simulink model "MultirotorSimPx4v1_8FPHTFullGainMatrix"  (R2020b)
settings: Solver=VariableStepAuto  StartTime=0.0  StopTime=Simulation.T_END  MaxStep=Simulation.TS_MAX  RelTol=1e-3  EnableMultiTasking=on
PreLoadFcn:
  | % InitializeParameters;
undefined symbols (not defined in the file): Aero, Ctrl, Initial, Motor, Uav, Wind
libraries: QuaternionLibrary x10, simulink_extras x2, cstblocks x1
(part 1 of 2)
settings Model: Creator=jban039  LastModifiedBy=jeremie
settings DataIOCC: Decimation=10  ExternalInput=getinputstruct(op1(2))  InitialState=getstatestruct(op)  SaveFormat=StructureWithTime  OutputTimes=Simulation.T_OUT
settings OptimizationCC: LifeSpan=inf
settings DebuggingCC: ReadBeforeWriteMsg=DisableAll  WriteAfterWriteMsg=DisableAll  WriteAfterReadMsg=DisableAll  MultiTaskDSMMsg=none  UnconnectedLineMsg=none  AllowSymbolicDim=off  SFUnexpectedBacktrackingDiag=warning  SFNoUnconditionalDefaultTransitionDiag=warning  SFExecutionAtInitializationDiag=none  ArithmeticOperatorsInVariantConditions=warning
settings ModelReferenceCC: UpdateModelReferenceTargets=IfOutOfDate  ModelReferenceMinAlgLoopOccurrences=on  PropagateSignalLabelsOutOfModel=off
settings SFSimCC: SFSimEcho=off  SimUseLocalCustomCode=off  CustomCodeUndefinedFunction=UseInterfaceOnly
settings RTWCC: RTWUseLocalCustomCode=off
settings CodeAppCC: StateflowObjectComments=on
settings GRTTargetCC: TargetLangStandard=C89/C90 (ANSI)
settings ConfigComp: CovMetricSettings=dw  CovSaveCumulativeToWorkspaceVar=on  CovSaveSingleToWorkspaceVar=on  CovExternalEMLEnable=off

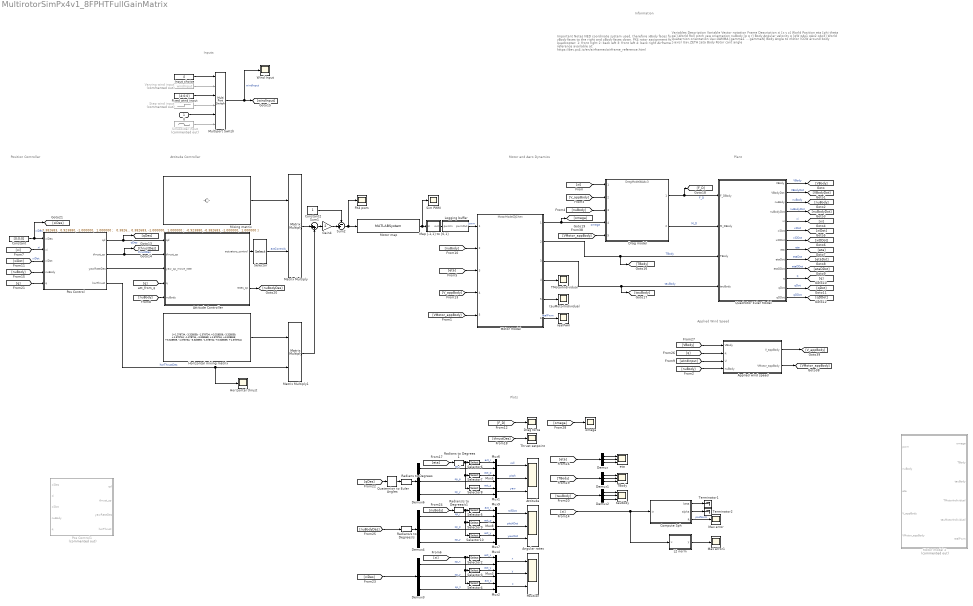
== system MultirotorSimPx4v1_8FPHTFullGainMatrix ==
  note: Plots
  note: Inputs
  note: Motor and Aero Dynamics
  note: Plant
  note: Attitude Controller
  note: Position Controller
  note: Applied Wind Speed
  note: Important Notes
      |
      | NED coordinate system used, therefore xBody faces forward, yBody faces to the right and zBody faces down.
      | PX4 rotor assignment for quadcopter:
      | 1: front right
      | 2: back left
      | 3: front left
      | 4: back right
      | Airframe reference available at:
      | https://dev.px4.io/en/airframes/airframe_reference.html
  note: Information
  note: Variables Description
      |
      | Variable
      | Vector notation
      | Frame
      | Description
      |
      | xi
      | [x y z]
      | World
      | Position
      |
      | eta
      | [phi theta psi]
      | World
      | Roll pitch yaw orientation
      |
      | nuBody
      | [p q r]
      | Body
      | Angular velocity
      |
      | q
      | [qW qAx1 qAx2 qAx3]
      | World
      | Quaternion orientation
      |
      | Uav.GAMMA
      | [gamma1 ... gammaN]
      | Body
      | Angle to motor (CCW around body z-axis)
      |
      | Uav.ZETA
      | zeta
      | Body
      | Rotor cant angle
  U : Inport  PortDimensions=3
  Angular rates : Scope  NumInputPorts=3
  Applied wind speed : Subsystem
  Attitude : Scope  NumInputPorts=3
  Attitude Controller : Subsystem
      mask Display: fprintf('MC_ATT_CONTROL\n\nCONTINUOUS')
  Compute Sph : MATLAB Function  TreatAsAtomicUnit=on
  Constant : Constant  Value=[0;0;0]
  Constant2 : Constant
  Demux{,1..4,6} (6 alike) : Demux  Outputs=3
  Drag force : Scope
  Drag model : ModelReference  ModelNameDialog=DragModelAIAAv3  SimulationMode=Normal  ModelReferenceVersion=5.2
  Fixed wind input : Constant  Value=[4;0;0]
  Gain4 : Gain  Gain=2
  Horizontal mixing matrix : Constant  Value=|
      | [+1.378734, -3.328559;
      |  -1.378734, +3.328559;
      |  -3.328559, +1.378734;
      |  -1.378734, -3.328559;
      |  +1.378734, +3.328559;
      |  +3.328559, -1.378734;
      |  -3.328559, -1.378734;
      |  +3.328559, +1.378734]
  Horizontal thrust : Scope
  Input choice : Constant  Value=4
  L2 norm : MATLAB Function  TreatAsAtomicUnit=on
  Logging buffer : Subsystem
  Map [-1,1] to [0,1] : Subsystem
  Matrix Multiply : Product  Multiplication=Matrix(*)
  Matrix Multiply1 : Product  Multiplication=Matrix(*)
  Max error : Scope
  Max error1 : Scope
  Mixing matrix : Constant  Value=|
      | [-0.382683,  0.923880, -1.000000,  1.000000 ;
      |   0.382683, -0.923880, -1.000000,  1.000000 ;
      |  -0.923880,  0.382683,  1.000000,  1.000000 ;
      |  -0.382683, -0.923880,  1.000000,  1.000000 ;
      |   0.382683,  0.923880,  1.000000,  1.000000 ;
      |   0.923880, -0.382683,  1.000000,  1.000000 ;
      |   0.923880,  0.382683, -1.000000,  1.000000 ;
      |  -0.923880, -0.382683, -1.000000,  1.000000 ]
  Motor map : MATLABSystem  System=MotorMap  airframeConfig=5  SimulateUsing=Code generation
      mask Type: MotorMap
      mask Display:
      | disp(['MOTOR' char(10) 'MAP' char(10) 'octa_x']);
      | port_label('input',1,'px4PWM');
      | port_label('output',1,'simPWM');
  Motor model : ModelReference  ModelNameDialog=MotorModelZJChen  SimulationMode=Normal  ModelReferenceVersion=5.6
  Motor model 2 : Subsystem  Commented=on
  Multiport Switch : MultiPortSwitch  Inputs=5
  Mux{1..9} (9 alike) : Mux  Inputs=2
  PX4 pwm : Scope
  Pos Control : Subsystem
      mask Display: fprintf('POS CONTROL\n\nFPHT\n\nCONTINUOUS')
  Pos Control1 : Subsystem  Commented=on
      mask Display: fprintf('POS CONTROL\n\nFPHT\n\nCONTINUOUS')
  Position : Scope  NumInputPorts=3
  Quadrotor Euler Model : Subsystem
  Quaternion to Euler Angles : QuaternionLibrary/Quaternion to Euler Angles
  "Radians to Degrees " : QuaternionLibrary/Radians to Degrees   SystemSampleTime=-1  VariantActivationTime=update diagram  Latency=0  AutoFrameSizeCalculation=off
  Radians to Degrees 1 : QuaternionLibrary/Radians to Degrees   SystemSampleTime=-1  VariantActivationTime=update diagram  Latency=0  AutoFrameSizeCalculation=off
  Radians/s to Degrees/s : QuaternionLibrary/Radians//s to Degrees//s  SystemSampleTime=-1  VariantActivationTime=update diagram  Latency=0  AutoFrameSizeCalculation=off
  Radians/s to Degrees/s1 : QuaternionLibrary/Radians//s to Degrees//s  SystemSampleTime=-1  VariantActivationTime=update diagram  Latency=0  AutoFrameSizeCalculation=off
  Selector : Selector  InputPortWidth=8  IndexOptions=Index vector (dialog)  Indices=[1:4]  OutputSizes=1
  Selector10 : Selector  InputPortWidth=3  IndexOptions=Index vector (dialog)  Indices=3  OutputSizes=1
  Selector2 : Selector  InputPortWidth=3  IndexOptions=Index vector (dialog)  Indices=1  OutputSizes=1
  Selector3 : Selector  InputPortWidth=3  IndexOptions=Index vector (dialog)  Indices=2  OutputSizes=1
  Selector4 : Selector  InputPortWidth=3  IndexOptions=Index vector (dialog)  Indices=3  OutputSizes=1
  Selector5 : Selector  InputPortWidth=3  IndexOptions=Index vector (dialog)  Indices=1  OutputSizes=1
  Selector6 : Selector  InputPortWidth=3  IndexOptions=Index vector (dialog)  Indices=1  OutputSizes=1
  Selector7 : Selector  InputPortWidth=3  IndexOptions=Index vector (dialog)  Indices=2  OutputSizes=1
  Selector8 : Selector  InputPortWidth=3  IndexOptions=Index vector (dialog)  Indices=3  OutputSizes=1
  Selector9 : Selector  InputPortWidth=3  IndexOptions=Index vector (dialog)  Indices=2  OutputSizes=1
  Sim PWM : Scope
  Sinusoidal input : Sin  Commented=on  Amplitude=Wind.Ampl  Bias=Wind.Bias  Frequency=Wind.Freq  SampleTime=0
  Step wind input : Step  Commented=on  Time=Wind.StepTime  Before=Wind.StepInit  After=Wind.StepFinal  SampleTime=0
  Sum1 : Sum  Inputs=|++
  Sum2 : Sum  Inputs=-+|
  TBody : Scope  NumInputPorts=3
  TMotorIndividual : Scope
  Terminator1 : Terminator
  Terminator2 : Terminator
  Thrust setpoint : Scope
  Varying wind input : FromWorkspace  Commented=on  VariableName=windInput
  Wind Input : Scope
  eta : Scope  NumInputPorts=3
  omega : Scope
  realPwm : Scope
  tauBody : Scope  NumInputPorts=3
  tauMotorIndividual : Scope
  wires:
  Motor model/1 -> Drag model/4, [omega]  "omega"
  Motor model/2 -> [TBody], Quadrotor Euler Model/3(TBody)  "TBody"
  Drag model/2 -> Quadrotor Euler Model/2(M_DBody)  "M_D"
  Quadrotor Euler Model/1(VBody) -> [VBody]  "VBody"
  Quadrotor Euler Model/2(VBodyDot) -> [VBodyDot]  "VBodyDot"
  Quadrotor Euler Model/3(nuBody) -> [nuBody]  "nuBody"
  Quadrotor Euler Model/4(nuBodyDot) -> [nuBodyDot]  "nuBodyDot"
  Quadrotor Euler Model/5(xi) -> [xi]  "xi"
  Quadrotor Euler Model/6(xiDot) -> [xiDot]  "xiDot"
  Quadrotor Euler Model/7(xiDDot) -> [xiDDot]  "xiDDot"
  Quadrotor Euler Model/8(eta) -> [eta]  "eta"
  Quadrotor Euler Model/9(etaDot) -> [etaDot]  "etaDot"
  Quadrotor Euler Model/10(etaDDot) -> [etaDDot]  "etaDDot"
  [V_appBody] -> Drag model/2
  [nuBody] -> Motor model/2
  Quadrotor Euler Model/11(q) -> [q]  "q"
  Quadrotor Euler Model/12(qDot) -> [qDot]  "qDot"
  Quadrotor Euler Model/13(qDDot) -> [qDDot]  "qDDot"
  Drag model/1 -> Quadrotor Euler Model/1(F_DBody), [F_D]  "F_D"
  Logging buffer/1(pwmOut) -> Motor model/1  "pwm"
  Sum2/1 -> PX4 pwm/1, Motor map/1
  [nuBody] -> Drag model/3
  [eta] -> Motor model/3
  [V_appBody] -> Motor model/4
  Motor model/4 -> TMotorIndividual/1
  Motor model/5 -> tauMotorIndividual/1
  [xi] -> Drag model/1
  [VMotor_appBody] -> Motor model/5
  [VMotor_appBody] -> Drag model/5
  Pos Control/1(qd) -> Attitude Controller/1(qd), [qDes]  "qDes"
  Motor model/3 -> [tauBody], Quadrotor Euler Model/4(tauBody)  "tauBody"
  [VBody] -> Applied wind speed/1(VBody)
  [q] -> Applied wind speed/2(q)
  [windInput] -> Applied wind speed/3(U)
  Applied wind speed/1(V_appBody) -> [V_appBody]
  Applied wind speed/2(VMotor_appBody) -> [VMotor_appBody]
  [nuBody] -> Applied wind speed/4(nuBody)
  Motor model/6 -> realPwm/1  "realPwm"
  [nuBody] -> Attitude Controller/5(nuBody)
  Motor map/1 -> Sim PWM/1, Map [-1,1] to [0,1]/1(in)
  Map [-1,1] to [0,1]/1(out) -> Logging buffer/1(pwmIn)
  Selector/1 -> Matrix Multiply/2  "actControls"
  Mixing matrix/1 -> Matrix Multiply/1
  Attitude Controller/1(actuators_control) -> Selector/1
  Gain4/1 -> Sum2/2
  Constant2/1 -> Sum2/1
  Matrix Multiply/1 -> Sum1/1
  Pos Control/2(thrust_sp) -> Attitude Controller/2(thrust_sp), [thrustDes]  "thrustDes"
  Pos Control/3(yawRateDes) -> Attitude Controller/3(yaw_sp_move_rate)
  [xiDot] -> Pos Control/3(xiDot)  "xiDot"
  [xi] -> Pos Control/2(xi)  "xi"
  [nuBody] -> Pos Control/4(nuBody)
  Constant/1 -> [xiDes], Pos Control/1(xiDes)  "xiDes"
  Attitude Controller/2(rates_sp) -> [nuBodyDes]
  Matrix Multiply1/1 -> Sum1/2
  Horizontal mixing matrix/1 -> Matrix Multiply1/1
  Pos Control/4(horThrust) -> Horizontal thrust/1, Matrix Multiply1/2  "horThrustDes"
  [q] -> Attitude Controller/4(q)
  [q] -> Pos Control/5(q)
  Sum1/1 -> Gain4/1
  Mux7/1 -> Angular rates/3  "yawDot"
  [nuBody] -> Radians/s to Degrees/s1/1
  Radians/s to Degrees/s1/1 -> Selector5/1, Selector9/1, Selector10/1
  Radians/s to Degrees/s/1 -> Demux4/1
  Mux8/1 -> Angular rates/2  "pitchDot"
  Mux9/1 -> Angular rates/1  "rollDot"
  Selector10/1 -> Mux7/1  "act_y"
  Demux4/2 -> Mux8/2  "sp_p"
  Demux4/1 -> Mux9/2  "sp_r"
  [nuBodyDes] -> Radians/s to Degrees/s/1
  Selector9/1 -> Mux8/1  "act_p"
  Selector5/1 -> Mux9/1  "act_r"
  Demux4/3 -> Mux7/2  "sp_y"
  Mux2/1 -> Position/3  "z"
  [xi] -> Selector2/1, Selector3/1, Selector4/1
  [xiDes] -> Demux3/1
  Mux3/1 -> Position/2  "y"
  Mux4/1 -> Position/1  "x"
  Selector4/1 -> Mux2/1  "act_z"
  Demux3/2 -> Mux3/2  "sp_y"
  Demux3/1 -> Mux4/2  "sp_x"
  Selector3/1 -> Mux3/1  "act_y"
  Selector2/1 -> Mux4/1  "act_x"
  Demux3/3 -> Mux2/2  "sp_z"
  L2 norm/1(y) -> Max error1/1
  [F_D] -> Drag force/1
  Compute Sph/3(R) -> Max error/1  "posNorm"
  Compute Sph/2(alpha) -> Terminator2/1
  Compute Sph/1(beta) -> Terminator1/1
  Demux2/3 -> tauBody/3
  Demux2/2 -> tauBody/2
  [tauBody] -> Demux2/1
  Demux2/1 -> tauBody/1
  Demux1/1 -> TBody/1
  [TBody] -> Demux1/1
  Demux1/2 -> TBody/2
  Demux1/3 -> TBody/3
  [thrustDes] -> Thrust setpoint/1
  Demux6/3 -> Mux1/2  "sp_y"
  Selector6/1 -> Mux6/1  "act_r"
  Selector7/1 -> Mux5/1  "act_p"
  Quaternion to Euler Angles/1 -> "Radians to Degrees "/1
  Demux6/1 -> Mux6/2  "sp_r"
  Demux6/2 -> Mux5/2  "sp_p"
  Selector8/1 -> Mux1/1  "act_y"
  [qDes] -> Quaternion to Euler Angles/1
  Mux6/1 -> Attitude/1  "roll"
  Mux5/1 -> Attitude/2  "pitch"
  "Radians to Degrees "/1 -> Demux6/1
  Radians to Degrees 1/1 -> Selector8/1, Selector7/1, Selector6/1
  [eta] -> Radians to Degrees 1/1
  Mux1/1 -> Attitude/3  "yaw"
  Demux/3 -> eta/3
  Demux/2 -> eta/2
  Demux/1 -> eta/1
  [eta] -> Demux/1
  [xi] -> Compute Sph/1(in), L2 norm/1(u)
  Sinusoidal input/1 -> Multiport Switch/6
  U/1 -> Multiport Switch/5
  Input choice/1 -> Multiport Switch/1
  Step wind input/1 -> Multiport Switch/4
  Multiport Switch/1 -> [windInput], Wind Input/1  "windInput"
  Fixed wind input/1 -> Multiport Switch/3
  Varying wind input/1 -> Multiport Switch/2
  [omega] -> omega/1

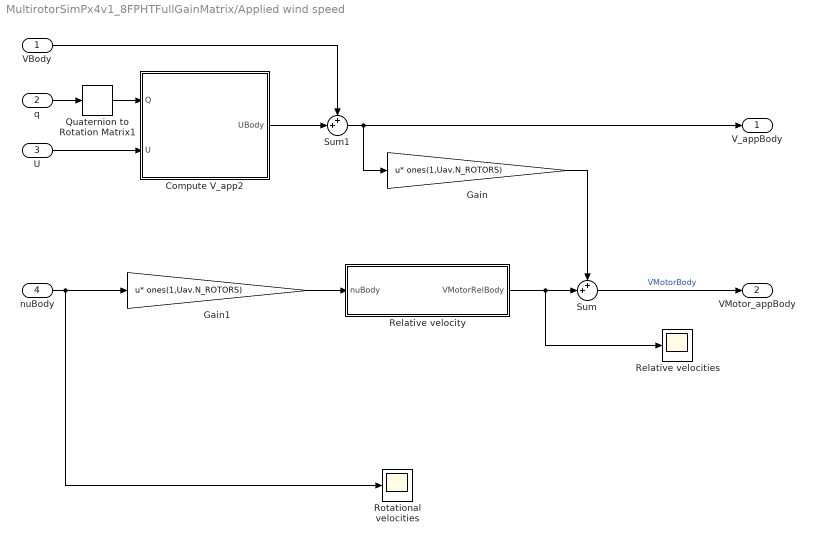
== system MultirotorSimPx4v1_8FPHTFullGainMatrix/Applied wind speed ==
  VBody : Inport  Unit=m/s
  q : Inport  Port=2
  U : Inport  Port=3  Unit=m/s
  nuBody : Inport  Port=4  Unit=rad/s
  Compute V_app2 : MATLAB Function  TreatAsAtomicUnit=on
  Gain : Gain  Gain=ones(1,Uav.N_ROTORS)  Multiplication=Matrix(u*K)
  Gain1 : Gain  Gain=ones(1,Uav.N_ROTORS)  Multiplication=Matrix(u*K)
  Quaternion to Rotation Matrix1 : QuaternionLibrary/Quaternion to Rotation Matrix
  Relative velocities : Scope
  Relative velocity : MATLAB Function  TreatAsAtomicUnit=on
  Rotational velocities : Scope
  Sum : Sum  Inputs=++|
  Sum1 : Sum  Inputs=++|
  V_appBody : Outport  Unit=m/s  VectorParamsAs1DForOutWhenUnconnected=off
  VMotor_appBody : Outport  Port=2  Unit=m/s  PortDimensions=[3,Uav.N_ROTORS]  VectorParamsAs1DForOutWhenUnconnected=off
  wires:
  U/1 -> Compute V_app2/2(U)
  Sum/1 -> VMotor_appBody/1  "VMotorBody"
  Quaternion to Rotation Matrix1/1 -> Compute V_app2/1(Q)
  nuBody/1 -> Gain1/1, Rotational velocities/1
  Gain/1 -> Sum/1
  VBody/1 -> Sum1/1
  q/1 -> Quaternion to Rotation Matrix1/1
  Relative velocity/1(VMotorRelBody) -> Relative velocities/1, Sum/2
  Compute V_app2/1(UBody) -> Sum1/2
  Sum1/1 -> Gain/1, V_appBody/1
  Gain1/1 -> Relative velocity/1(nuBody)

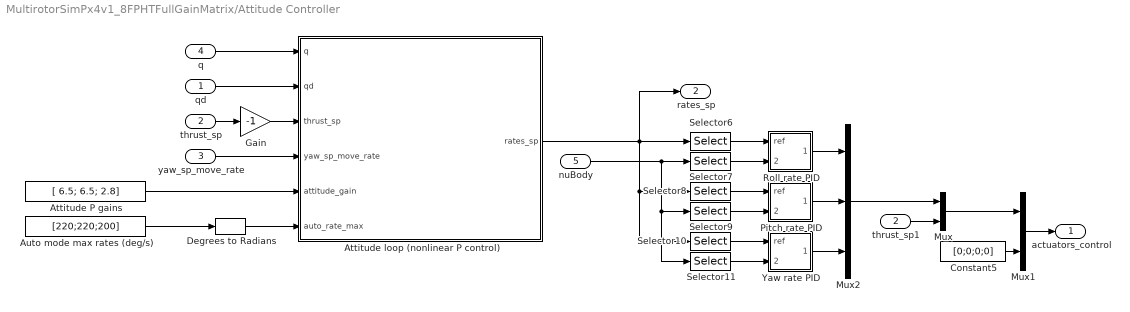
== system MultirotorSimPx4v1_8FPHTFullGainMatrix/Attitude Controller ==
  qd : Inport
  thrust_sp : Inport  Port=2  PortDimensions=1
  yaw_sp_move_rate : Inport  Port=3
  q : Inport  Port=4
  nuBody : Inport  Port=5
  Attitude P gains : Constant  Value=[ 6.5; 6.5; 2.8]
  Attitude loop (nonlinear P control) : MATLAB Function  TreatAsAtomicUnit=on
  Auto mode max rates (deg/s) : Constant  Value=[220;220;200]
  Constant5 : Constant  Value=[0;0;0;0]
  Degrees to Radians : simulink_extras/Transformations/Degrees to Radians
  Gain : Gain  Gain=-1
  Mux : Mux  Inputs=2
  Mux1 : Mux  Inputs=2
  Mux2 : Mux  Inputs=3
  Pitch rate PID : Subsystem  mask{PID_P=0.15, PID_I=0.05, PID_D=0.003, PID_FC=30, PID_I_STATENAME='AttRatePID_I_pitch', PID_D_STATENAME='AttRatePID_D_pitch'}
      mask prompts: PID_P "P gain"; PID_I "I gain"; PID_D "D gain"; PID_FC "D filter cutoff (Hz)"; PID_I_STATENAME "Integartor state name"; PID_D_STATENAME "D filter state name"
      mask DialogControl DescGroupVar Prompt: PID Controller with Second Order Derivative Filter
      mask DialogControl DescTextVar Prompt: The derivative gain is applied on the derivative of y rather than that of the error (r-y).
      mask Display:
      | disp('PID(s)')
      | port_label('input', 1, 'r')
      | port_label('input', 2, 'y')
      | text(1,0,'2^{nd}','horizontalAlignment','right','interpreter','tex','verticalAlignment','bottom')
  Roll rate PID : Subsystem  mask{PID_P=0.15, PID_I=0.05, PID_D=0.003, PID_FC=30, PID_I_STATENAME='AttRatePID_I_roll', PID_D_STATENAME='AttRatePID_D_roll'}
      mask prompts: PID_P "P gain"; PID_I "I gain"; PID_D "D gain"; PID_FC "D filter cutoff (Hz)"; PID_I_STATENAME "Integartor state name"; PID_D_STATENAME "D filter state name"
      mask DialogControl DescGroupVar Prompt: PID Controller with Second Order Derivative Filter
      mask DialogControl DescTextVar Prompt: The derivative gain is applied on the derivative of y rather than that of the error (r-y).
      mask Display:
      | disp('PID(s)')
      | port_label('input', 1, 'r')
      | port_label('input', 2, 'y')
      | text(1,0,'2^{nd}','horizontalAlignment','right','interpreter','tex','verticalAlignment','bottom')
  Selector10 : Selector  InputPortWidth=3  IndexOptions=Index vector (dialog)  Indices=3  OutputSizes=1
  Selector11 : Selector  InputPortWidth=3  IndexOptions=Index vector (dialog)  Indices=3  OutputSizes=1
  Selector6 : Selector  InputPortWidth=3  IndexOptions=Index vector (dialog)  Indices=1  OutputSizes=1
  Selector7 : Selector  InputPortWidth=3  IndexOptions=Index vector (dialog)  Indices=1  OutputSizes=1
  Selector8 : Selector  InputPortWidth=3  IndexOptions=Index vector (dialog)  Indices=2  OutputSizes=1
  Selector9 : Selector  InputPortWidth=3  IndexOptions=Index vector (dialog)  Indices=2  OutputSizes=1
  Yaw rate PID : Subsystem  mask{PID_P=0.2, PID_I=0.1, PID_D=0, PID_FC=30, PID_I_STATENAME='AttRatePID_I_yaw', PID_D_STATENAME='AttRatePID_D_yaw'}
      mask prompts: PID_P "P gain"; PID_I "I gain"; PID_D "D gain"; PID_FC "D filter cutoff (Hz)"; PID_I_STATENAME "Integartor state name"; PID_D_STATENAME "D filter state name"
      mask DialogControl DescGroupVar Prompt: PID Controller with Second Order Derivative Filter
      mask DialogControl DescTextVar Prompt: The derivative gain is applied on the derivative of y rather than that of the error (r-y).
      mask Display:
      | disp('PID(s)')
      | port_label('input', 1, 'r')
      | port_label('input', 2, 'y')
      | text(1,0,'2^{nd}','horizontalAlignment','right','interpreter','tex','verticalAlignment','bottom')
  thrust_sp1 : InportShadow  Port=2  PortDimensions=1
  actuators_control : Outport  PortDimensions=8  VectorParamsAs1DForOutWhenUnconnected=off
  rates_sp : Outport  Port=2  VectorParamsAs1DForOutWhenUnconnected=off
  wires:
  thrust_sp1/1 -> Mux/2
  Gain/1 -> Attitude loop (nonlinear P control)/3(thrust_sp)
  Attitude loop (nonlinear P control)/1(rates_sp) -> rates_sp/1, Selector10/1, Selector8/1, Selector6/1
  thrust_sp/1 -> Gain/1
  Mux1/1 -> actuators_control/1
  Constant5/1 -> Mux1/2
  Mux/1 -> Mux1/1
  yaw_sp_move_rate/1 -> Attitude loop (nonlinear P control)/4(yaw_sp_move_rate)
  Degrees to Radians/1 -> Attitude loop (nonlinear P control)/6(auto_rate_max)
  Auto mode max rates (deg/s)/1 -> Degrees to Radians/1
  Attitude P gains/1 -> Attitude loop (nonlinear P control)/5(attitude_gain)
  q/1 -> Attitude loop (nonlinear P control)/1(q)
  qd/1 -> Attitude loop (nonlinear P control)/2(qd)
  Yaw rate PID/1(Out) -> Mux2/3
  Roll rate PID/1(Out) -> Mux2/1
  Pitch rate PID/1(Out) -> Mux2/2
  Mux2/1 -> Mux/1
  Selector6/1 -> Roll rate PID/1(ref)
  Selector7/1 -> Roll rate PID/2(meas)
  Selector8/1 -> Pitch rate PID/1(ref)
  Selector10/1 -> Yaw rate PID/1(ref)
  Selector11/1 -> Yaw rate PID/2(meas)
  Selector9/1 -> Pitch rate PID/2(meas)
  nuBody/1 -> Selector11/1, Selector9/1, Selector7/1

== system MultirotorSimPx4v1_8FPHTFullGainMatrix/Logging buffer ==
  pwmIn : Inport
  pwmOut : Outport  VectorParamsAs1DForOutWhenUnconnected=off
  wires:
  pwmIn/1 -> pwmOut/1

== system MultirotorSimPx4v1_8FPHTFullGainMatrix/Map [-1,1] to [0,1] ==
  in : Inport
  Constant : Constant
  Gain4 : Gain  Gain=0.5
  Sum : Sum  Inputs=++|
  out : Outport  VectorParamsAs1DForOutWhenUnconnected=off
  wires:
  Sum/1 -> Gain4/1
  Gain4/1 -> out/1
  in/1 -> Sum/2
  Constant/1 -> Sum/1

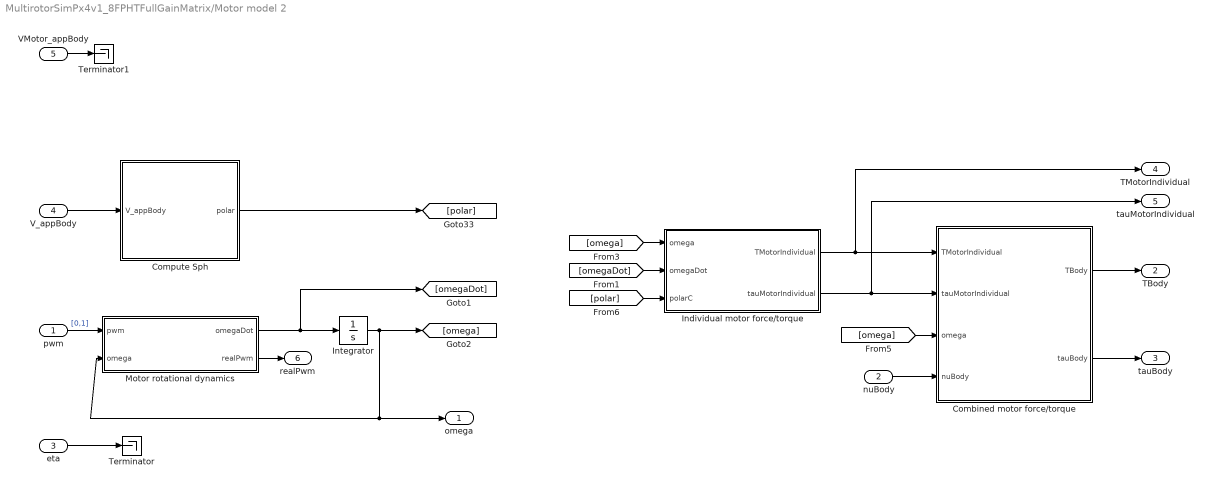
== system MultirotorSimPx4v1_8FPHTFullGainMatrix/Motor model 2 ==
  pwm : Inport  PortDimensions=Uav.N_ROTORS
  nuBody : Inport  Port=2  Unit=rad/s  PortDimensions=3
  eta : Inport  Port=3  Unit=rad  PortDimensions=3
  V_appBody : Inport  Port=4  Unit=m/s  PortDimensions=3
  VMotor_appBody : Inport  Port=5  Unit=m/s  PortDimensions=[3,Uav.N_ROTORS]
  Combined motor force/torque : MATLAB Function  TreatAsAtomicUnit=on
  Compute Sph : MATLAB Function  TreatAsAtomicUnit=on
  Individual motor force/torque : MATLAB Function  TreatAsAtomicUnit=on
  Integrator : Integrator  InitialCondition=Initial.OMEGA  LimitOutput=on  LowerSaturationLimit=zeros(size(Initial.OMEGA))  ContinuousStateAttributes='omega'
  Motor rotational dynamics : MATLAB Function  TreatAsAtomicUnit=on
  Terminator : Terminator
  Terminator1 : Terminator
  omega : Outport  Unit=rad/s  VectorParamsAs1DForOutWhenUnconnected=off
  TBody : Outport  Port=2  Unit=N  VectorParamsAs1DForOutWhenUnconnected=off
  tauBody : Outport  Port=3  Unit=N*m  VectorParamsAs1DForOutWhenUnconnected=off
  TMotorIndividual : Outport  Port=4  Unit=N  PortDimensions=[3,Uav.N_ROTORS]  VectorParamsAs1DForOutWhenUnconnected=off
  tauMotorIndividual : Outport  Port=5  Unit=N  PortDimensions=[3,Uav.N_ROTORS]  VectorParamsAs1DForOutWhenUnconnected=off
  realPwm : Outport  Port=6  VectorParamsAs1DForOutWhenUnconnected=off
  wires:
  [omegaDot] -> Individual motor force/torque/2(omegaDot)
  Compute Sph/1(polar) -> [polar]
  pwm/1 -> Motor rotational dynamics/1(pwm)  "[0,1]"
  [omega] -> Combined motor force/torque/3(omega)
  Combined motor force/torque/1(TBody) -> TBody/1
  [omega] -> Individual motor force/torque/1(omega)
  eta/1 -> Terminator/1
  V_appBody/1 -> Compute Sph/1(V_appBody)
  Individual motor force/torque/1(TMotorIndividual) -> Combined motor force/torque/1(TMotorIndividual), TMotorIndividual/1
  Motor rotational dynamics/1(omegaDot) -> [omegaDot], Integrator/1
  Integrator/1 -> [omega], Motor rotational dynamics/2(omega), omega/1
  Individual motor force/torque/2(tauMotorIndividual) -> tauMotorIndividual/1, Combined motor force/torque/2(tauMotorIndividual)
  nuBody/1 -> Combined motor force/torque/4(nuBody)
  Combined motor force/torque/2(tauBody) -> tauBody/1
  Motor rotational dynamics/2(realPwm) -> realPwm/1
  VMotor_appBody/1 -> Terminator1/1
  [polar] -> Individual motor force/torque/3(polarC)

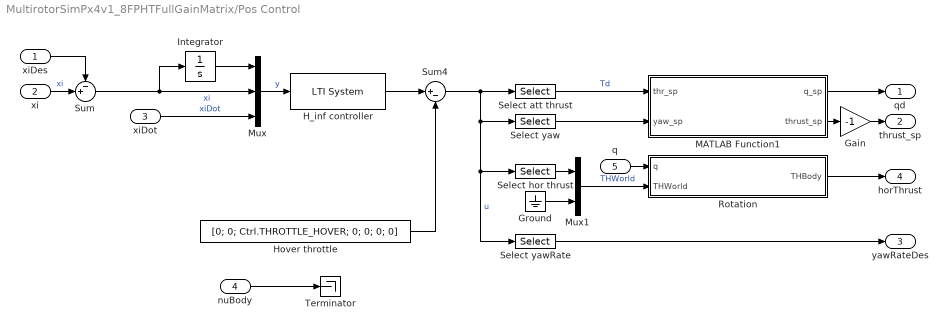
== system MultirotorSimPx4v1_8FPHTFullGainMatrix/Pos Control ==
  xiDes : Inport  Unit=m  PortDimensions=3
  xi : Inport  Port=2  Unit=m  PortDimensions=3
  xiDot : Inport  Port=3  Unit=m/s  PortDimensions=3
  nuBody : Inport  Port=4  Unit=rad/s
  q : Inport  Port=5
  Gain : Gain  Gain=-1
  Ground : Ground
  H_inf controller : cstblocks/LTI System  sys=Ctrl.K  IC=[]
  Hover throttle : Constant  Value=[0; 0; Ctrl.THROTTLE_HOVER; 0; 0; 0; 0]
  Integrator : Integrator
  MATLAB Function1 : MATLAB Function  TreatAsAtomicUnit=on
  Mux : Mux  Inputs=3
  Mux1 : Mux  Inputs=2
  Rotation : Subsystem
  Select att thrust : Selector  InputPortWidth=size(Ctrl.K.C, 1)  IndexOptions=Index vector (dialog)  Indices=[1:3]  OutputSizes=1
  Select hor thrust : Selector  InputPortWidth=size(Ctrl.K.C, 1)  IndexOptions=Index vector (dialog)  Indices=[4:5]  OutputSizes=1
  Select yaw : Selector  InputPortWidth=size(Ctrl.K.C, 1)  IndexOptions=Index vector (dialog)  Indices=[6]  OutputSizes=1
  Select yawRate : Selector  InputPortWidth=size(Ctrl.K.C, 1)  IndexOptions=Index vector (dialog)  Indices=[7]  OutputSizes=1
  Sum : Sum  Inputs=-+|
  Sum4 : Sum  Inputs=|+-
  Terminator : Terminator
  qd : Outport  VectorParamsAs1DForOutWhenUnconnected=off
  thrust_sp : Outport  Port=2  VectorParamsAs1DForOutWhenUnconnected=off
  yawRateDes : Outport  Port=3  Unit=rad/s  VectorParamsAs1DForOutWhenUnconnected=off
  horThrust : Outport  Port=4  PortDimensions=2  VectorParamsAs1DForOutWhenUnconnected=off
  wires:
  Select yawRate/1 -> yawRateDes/1
  nuBody/1 -> Terminator/1
  Rotation/1(THBody) -> horThrust/1
  Select yaw/1 -> MATLAB Function1/2(yaw_sp)
  MATLAB Function1/1(q_sp) -> qd/1
  MATLAB Function1/2(thrust_sp) -> Gain/1
  Select att thrust/1 -> MATLAB Function1/1(thr_sp)  "Td"
  Sum/1 -> Mux/2, Integrator/1  "xi"
  q/1 -> Rotation/1(q)
  Mux1/1 -> Rotation/2(THWorld)  "THWorld"
  Mux/1 -> H_inf controller/1  "y"
  Hover throttle/1 -> Sum4/2
  Sum4/1 -> Select yaw/1, Select yawRate/1, Select hor thrust/1, Select att thrust/1  "u"
  Gain/1 -> thrust_sp/1
  xiDes/1 -> Sum/1
  xi/1 -> Sum/2  "xi"
  Integrator/1 -> Mux/1
  xiDot/1 -> Mux/3  "xiDot"
  H_inf controller/1 -> Sum4/1
  Select hor thrust/1 -> Mux1/1
  Ground/1 -> Mux1/2

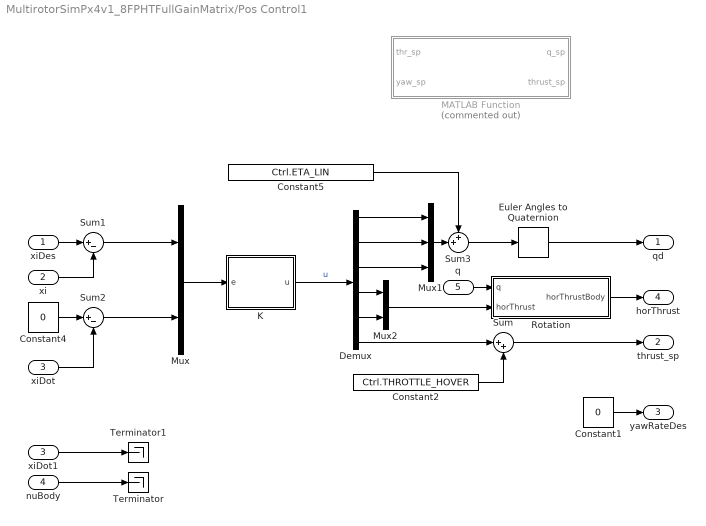
== system MultirotorSimPx4v1_8FPHTFullGainMatrix/Pos Control1 ==
  xiDes : Inport  Unit=m  PortDimensions=3
  xi : Inport  Port=2  Unit=m  PortDimensions=3
  xiDot : Inport  Port=3  Unit=m/s  PortDimensions=3
  nuBody : Inport  Port=4  Unit=rad/s
  q : Inport  Port=5
  Constant1 : Constant  Value=0
  Constant2 : Constant  Value=Ctrl.THROTTLE_HOVER
  Constant4 : Constant  Value=0
  Constant5 : Constant  Value=Ctrl.ETA_LIN
  Demux : Demux  Outputs=6
  Euler Angles to Quaternion : QuaternionLibrary/Euler Angles to Quaternion
  K : Subsystem
      mask Display:
      | text(0.5, 0.5, '\fontsize{30}K', 'horizontalAlignment', ...
      |     'center', 'verticalAlignment', 'middle', 'texmode', 'on')
  MATLAB Function : MATLAB Function  Commented=on  TreatAsAtomicUnit=on
  Mux : Mux  Inputs=2
  Mux1 : Mux  Inputs=3
  Mux2 : Mux  Inputs=2
  Rotation : Subsystem  VariantControl=HorThrustNoVertComp
  Sum : Sum  Inputs=|++
  Sum1 : Sum  Inputs=|+-
  Sum2 : Sum  Inputs=|+-
  Sum3 : Sum  Inputs=++|
  Terminator : Terminator
  Terminator1 : Terminator
  xiDot1 : InportShadow  Port=3  Unit=m/s  PortDimensions=3
  qd : Outport  VectorParamsAs1DForOutWhenUnconnected=off
  thrust_sp : Outport  Port=2  VectorParamsAs1DForOutWhenUnconnected=off
  yawRateDes : Outport  Port=3  Unit=rad/s  VectorParamsAs1DForOutWhenUnconnected=off
  horThrust : Outport  Port=4  PortDimensions=2  VectorParamsAs1DForOutWhenUnconnected=off
  wires:
  Mux1/1 -> Sum3/2
  Constant5/1 -> Sum3/1
  Demux/2 -> Mux1/2
  Constant2/1 -> Sum/2
  Sum/1 -> thrust_sp/1
  Rotation/1(" horThrustBody") -> horThrust/1
  q/1 -> Rotation/1("q ")
  Mux2/1 -> Rotation/2("horThrust ")
  Demux/5 -> Mux2/2
  Demux/4 -> Mux2/1
  Demux/6 -> Sum/1
  Euler Angles to Quaternion/1 -> qd/1
  Sum3/1 -> Euler Angles to Quaternion/1
  Demux/1 -> Mux1/1
  Demux/3 -> Mux1/3
  K/1(u) -> Demux/1  "u"
  Mux/1 -> K/1(e)
  Sum2/1 -> Mux/2
  Constant4/1 -> Sum2/1
  xiDot/1 -> Sum2/2
  Sum1/1 -> Mux/1
  xiDot1/1 -> Terminator1/1
  nuBody/1 -> Terminator/1
  xiDes/1 -> Sum1/1
  xi/1 -> Sum1/2
  Constant1/1 -> yawRateDes/1

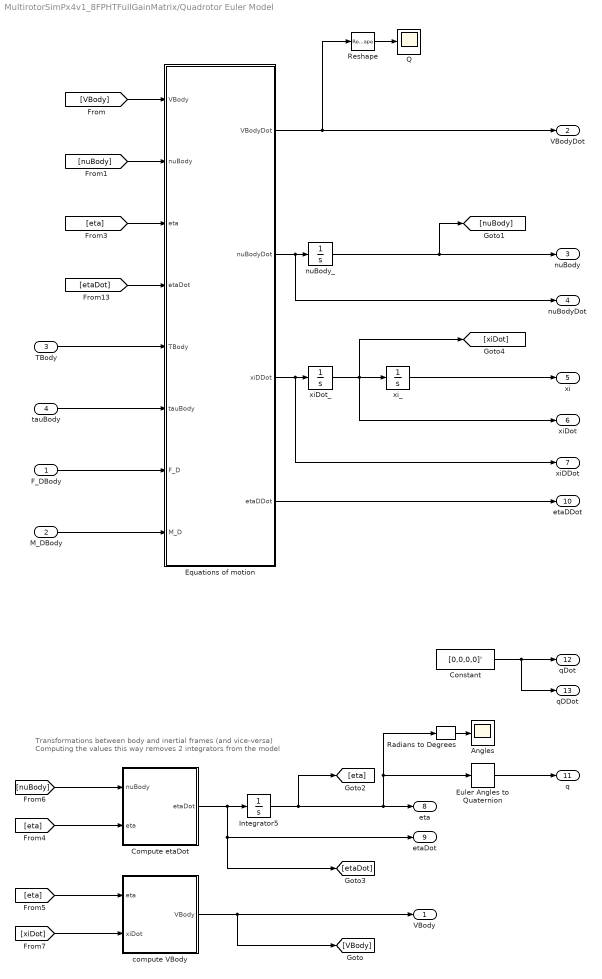
== system MultirotorSimPx4v1_8FPHTFullGainMatrix/Quadrotor Euler Model ==
  note: Transformations between body and inertial frames (and vice-versa)
      | Computing the values this way removes 2 integrators from the model
  F_DBody : Inport  Unit=N
  M_DBody : Inport  Port=2  Unit=N*m
  TBody : Inport  Port=3  Unit=N
  tauBody : Inport  Port=4  Unit=N*m
  Angles : Scope
  Compute etaDot : MATLAB Function  TreatAsAtomicUnit=on
  Constant : Constant  Value=[0,0,0,0]'
  Equations of motion : MATLAB Function  TreatAsAtomicUnit=on
  Euler Angles to Quaternion : QuaternionLibrary/Euler Angles to Quaternion
  Integrator5 : Integrator  InitialCondition=Initial.ETA  ContinuousStateAttributes='eta'
  Q : Scope
  Radians to Degrees : simulink_extras/Transformations/Radians to Degrees
  Reshape : Reshape  OutputDimensionality=Column vector (2-D)
  compute VBody : MATLAB Function  TreatAsAtomicUnit=on
  nuBody_ : Integrator  InitialCondition=Initial.NU_BODY  ContinuousStateAttributes='nuBody'
  xiDot_ : Integrator  InitialCondition=Initial.XI_DOT  ContinuousStateAttributes='xiDot'
  xi_ : Integrator  InitialCondition=Initial.XI  ContinuousStateAttributes='xi'
  VBody : Outport  Unit=m/s  VectorParamsAs1DForOutWhenUnconnected=off
  VBodyDot : Outport  Port=2  Unit=m/s^2  VectorParamsAs1DForOutWhenUnconnected=off
  nuBody : Outport  Port=3  Unit=rad/s  VectorParamsAs1DForOutWhenUnconnected=off
  nuBodyDot : Outport  Port=4  Unit=rad/s^2  VectorParamsAs1DForOutWhenUnconnected=off
  xi : Outport  Port=5  Unit=m  VectorParamsAs1DForOutWhenUnconnected=off
  xiDot : Outport  Port=6  Unit=m/s  VectorParamsAs1DForOutWhenUnconnected=off
  xiDDot : Outport  Port=7  Unit=m/s^2  VectorParamsAs1DForOutWhenUnconnected=off
  eta : Outport  Port=8  Unit=rad  VectorParamsAs1DForOutWhenUnconnected=off
  etaDot : Outport  Port=9  Unit=rad/s  VectorParamsAs1DForOutWhenUnconnected=off
  etaDDot : Outport  Port=10  Unit=rad/s^2  VectorParamsAs1DForOutWhenUnconnected=off
  q : Outport  Port=11  VectorParamsAs1DForOutWhenUnconnected=off
  qDot : Outport  Port=12  VectorParamsAs1DForOutWhenUnconnected=off
  qDDot : Outport  Port=13  VectorParamsAs1DForOutWhenUnconnected=off
  wires:
  Radians to Degrees/1 -> Angles/1
  Constant/1 -> qDot/1, qDDot/1
  Euler Angles to Quaternion/1 -> q/1
  Integrator5/1 -> [eta], eta/1, Euler Angles to Quaternion/1, Radians to Degrees/1
  Compute etaDot/1(etaDot) -> Integrator5/1, [etaDot], etaDot/1
  [eta] -> Compute etaDot/2(eta)
  compute VBody/1(VBody) -> [VBody], VBody/1
  [eta] -> compute VBody/1(eta)
  [nuBody] -> Compute etaDot/1(nuBody)
  [xiDot] -> compute VBody/2(xiDot)
  [etaDot] -> Equations of motion/4(etaDot)
  xiDot_/1 -> xiDot/1, [xiDot], xi_/1
  Reshape/1 -> Q/1
  Equations of motion/4(etaDDot) -> etaDDot/1
  [eta] -> Equations of motion/3(eta)
  Equations of motion/2(nuBodyDot) -> nuBodyDot/1, nuBody_/1
  nuBody_/1 -> nuBody/1, [nuBody]
  M_DBody/1 -> Equations of motion/8(M_D)
  F_DBody/1 -> Equations of motion/7(F_D)
  Equations of motion/3(xiDDot) -> xiDDot/1, xiDot_/1
  TBody/1 -> Equations of motion/5(TBody)
  tauBody/1 -> Equations of motion/6(tauBody)
  [VBody] -> Equations of motion/1(VBody)
  [nuBody] -> Equations of motion/2(nuBody)
  xi_/1 -> xi/1
  Equations of motion/1(VBodyDot) -> VBodyDot/1, Reshape/1

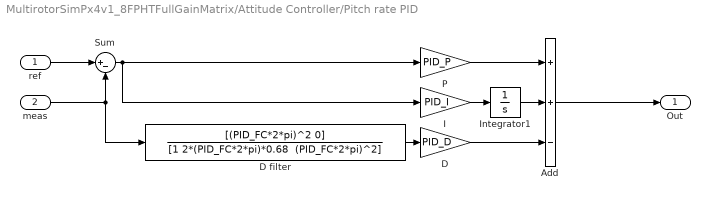
== system MultirotorSimPx4v1_8FPHTFullGainMatrix/Attitude Controller/Pitch rate PID ==
  ref : Inport
  meas : Inport  Port=2
  Add : Sum  Inputs=++-
  D : Gain  Gain=PID_D
  D filter : TransferFcn  Numerator=[(PID_FC*2*pi)^2 0]  Denominator="[1 2*(PID_FC*2*pi)*0.68  (PID_FC*2*pi)^2]"  ContinuousStateAttributes=PID_D_STATENAME
  I : Gain  Gain=PID_I
  Integrator1 : Integrator  LimitOutput=on  UpperSaturationLimit=0.3  LowerSaturationLimit=-0.3  ContinuousStateAttributes=PID_I_STATENAME
  P : Gain  Gain=PID_P
  Sum : Sum  Inputs=|+-
  Out : Outport  VectorParamsAs1DForOutWhenUnconnected=off
  wires:
  Add/1 -> Out/1
  P/1 -> Add/1
  Integrator1/1 -> Add/2
  D filter/1 -> D/1
  Sum/1 -> P/1, I/1
  D/1 -> Add/3
  I/1 -> Integrator1/1
  ref/1 -> Sum/1
  meas/1 -> D filter/1, Sum/2

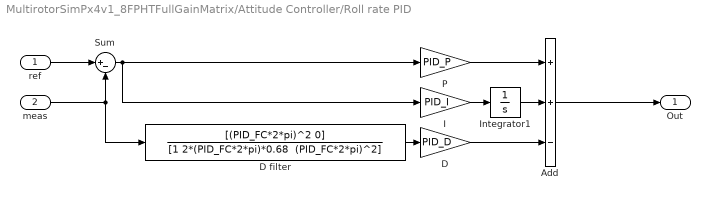
== system MultirotorSimPx4v1_8FPHTFullGainMatrix/Attitude Controller/Roll rate PID ==
  ref : Inport
  meas : Inport  Port=2
  Add : Sum  Inputs=++-
  D : Gain  Gain=PID_D
  D filter : TransferFcn  Numerator=[(PID_FC*2*pi)^2 0]  Denominator="[1 2*(PID_FC*2*pi)*0.68  (PID_FC*2*pi)^2]"  ContinuousStateAttributes=PID_D_STATENAME
  I : Gain  Gain=PID_I
  Integrator1 : Integrator  LimitOutput=on  UpperSaturationLimit=0.3  LowerSaturationLimit=-0.3  ContinuousStateAttributes=PID_I_STATENAME
  P : Gain  Gain=PID_P
  Sum : Sum  Inputs=|+-
  Out : Outport  VectorParamsAs1DForOutWhenUnconnected=off
  wires:
  meas/1 -> Sum/2, D filter/1
  ref/1 -> Sum/1
  I/1 -> Integrator1/1
  D/1 -> Add/3
  Sum/1 -> I/1, P/1
  D filter/1 -> D/1
  Integrator1/1 -> Add/2
  P/1 -> Add/1
  Add/1 -> Out/1

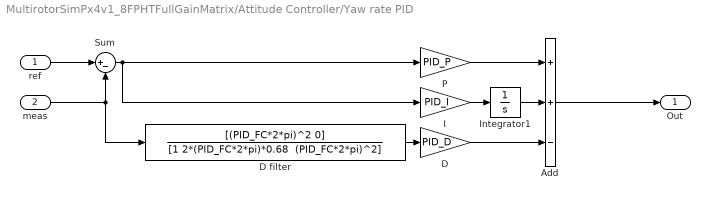
== system MultirotorSimPx4v1_8FPHTFullGainMatrix/Attitude Controller/Yaw rate PID ==
  ref : Inport
  meas : Inport  Port=2
  Add : Sum  Inputs=++-
  D : Gain  Gain=PID_D
  D filter : TransferFcn  Numerator=[(PID_FC*2*pi)^2 0]  Denominator="[1 2*(PID_FC*2*pi)*0.68  (PID_FC*2*pi)^2]"  ContinuousStateAttributes=PID_D_STATENAME
  I : Gain  Gain=PID_I
  Integrator1 : Integrator  LimitOutput=on  UpperSaturationLimit=0.3  LowerSaturationLimit=-0.3  ContinuousStateAttributes=PID_I_STATENAME
  P : Gain  Gain=PID_P
  Sum : Sum  Inputs=|+-
  Out : Outport  VectorParamsAs1DForOutWhenUnconnected=off
  wires:
  meas/1 -> Sum/2, D filter/1
  ref/1 -> Sum/1
  I/1 -> Integrator1/1
  D/1 -> Add/3
  Sum/1 -> I/1, P/1
  D filter/1 -> D/1
  Integrator1/1 -> Add/2
  P/1 -> Add/1
  Add/1 -> Out/1

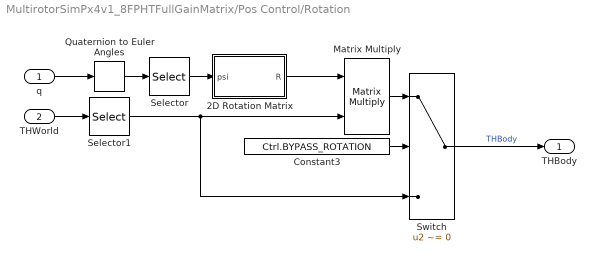
== system MultirotorSimPx4v1_8FPHTFullGainMatrix/Pos Control/Rotation ==
  q : Inport
  THWorld : Inport  Port=2
  2D Rotation Matrix : Subsystem
  Constant3 : Constant  Value=Ctrl.BYPASS_ROTATION
  Matrix Multiply : Product  Multiplication=Matrix(*)
  Quaternion to Euler Angles : QuaternionLibrary/Quaternion to Euler Angles
  Selector : Selector  InputPortWidth=3  IndexOptions=Index vector (dialog)  Indices=3  OutputSizes=1
  Selector1 : Selector  InputPortWidth=3  IndexOptions=Index vector (dialog)  Indices=[1 2]  OutputSizes=1
  Switch : Switch  Criteria=u2 ~= 0
  THBody : Outport  VectorParamsAs1DForOutWhenUnconnected=off
  wires:
  q/1 -> Quaternion to Euler Angles/1
  THWorld/1 -> Selector1/1
  Matrix Multiply/1 -> Switch/1
  Switch/1 -> THBody/1  "THBody"
  2D Rotation Matrix/1(R) -> Matrix Multiply/1
  Quaternion to Euler Angles/1 -> Selector/1
  Selector/1 -> 2D Rotation Matrix/1(psi)
  Constant3/1 -> Switch/2
  Selector1/1 -> Switch/3, Matrix Multiply/2

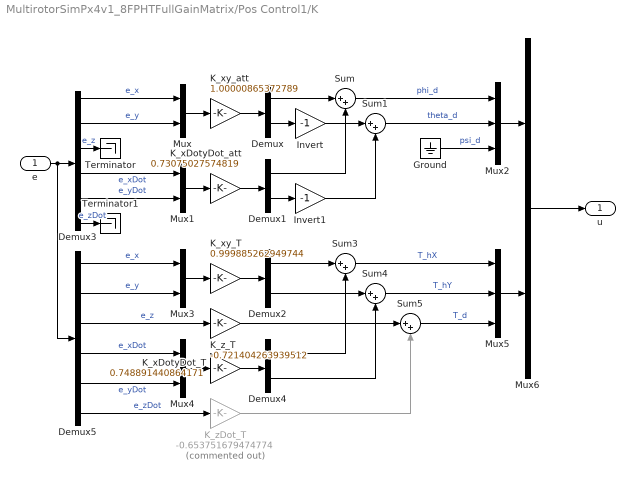
== system MultirotorSimPx4v1_8FPHTFullGainMatrix/Pos Control1/K ==
  e : Inport
  Demux{,1..2,4} (4 alike) : Demux  Outputs=2
  Demux3 : Demux  Outputs=6
  Demux5 : Demux  Outputs=6
  Ground : Ground
  Invert : Gain  Gain=-1
  Invert1 : Gain  Gain=-1
  K_xDotyDot_T : Gain  Gain=0.748891440864171
  K_xDotyDot_att : Gain  Gain=0.73075027574819
  K_xy_T : Gain  Gain=0.999885262949744
  K_xy_att : Gain  Gain=1.00000865372789
  K_zDot_T : Gain  Commented=on  Gain=-0.653751679474774
  K_z_T : Gain  Gain=-0.721404263939512
  Mux{,1,3..4,6} (5 alike) : Mux  Inputs=2
  Mux2 : Mux  Inputs=3
  Mux5 : Mux  Inputs=3
  Sum{,1,3..5} (5 alike) : Sum  Inputs=|++
  Terminator : Terminator
  Terminator1 : Terminator
  u : Outport  VectorParamsAs1DForOutWhenUnconnected=off
  wires:
  Mux6/1 -> u/1
  Demux3/1 -> Mux/1  "e_x"
  e/1 -> Demux5/1, Demux3/1
  Demux3/4 -> Mux1/1  "e_xDot"
  Demux3/5 -> Mux1/2  "e_yDot"
  Demux3/2 -> Mux/2  "e_y"
  Mux/1 -> K_xy_att/1
  K_xy_att/1 -> Demux/1
  Demux/1 -> Sum/1
  Demux/2 -> Invert/1
  K_xDotyDot_att/1 -> Demux1/1
  Mux1/1 -> K_xDotyDot_att/1
  Demux1/2 -> Invert1/1
  Demux1/1 -> Sum/2
  Demux4/1 -> Sum3/2
  K_z_T/1 -> Sum5/1
  K_zDot_T/1 -> Sum5/2
  Demux4/2 -> Sum4/2
  Mux4/1 -> K_xDotyDot_T/1
  K_xDotyDot_T/1 -> Demux4/1
  Demux2/2 -> Sum4/1
  Demux2/1 -> Sum3/1
  K_xy_T/1 -> Demux2/1
  Mux3/1 -> K_xy_T/1
  Demux5/2 -> Mux3/2  "e_y"
  Demux5/5 -> Mux4/2  "e_yDot"
  Demux5/3 -> K_z_T/1  "e_z"
  Demux5/6 -> K_zDot_T/1  "e_zDot"
  Demux5/4 -> Mux4/1  "e_xDot"
  Demux5/1 -> Mux3/1  "e_x"
  Sum/1 -> Mux2/1  "phi_d"
  Sum1/1 -> Mux2/2  "theta_d"
  Sum5/1 -> Mux5/3  "T_d"
  Sum4/1 -> Mux5/2  "T_hY"
  Sum3/1 -> Mux5/1  "T_hX"
  Mux2/1 -> Mux6/1
  Mux5/1 -> Mux6/2
  Demux3/3 -> Terminator/1  "e_z"
  Demux3/6 -> Terminator1/1  "e_zDot"
  Ground/1 -> Mux2/3  "psi_d"
  Invert1/1 -> Sum1/2
  Invert/1 -> Sum1/1

== system MultirotorSimPx4v1_8FPHTFullGainMatrix/Pos Control1/Rotation ==
  "q " : Inport
  "horThrust " : Inport  Port=2
  2D Rotation Matrix : Subsystem
  Matrix Multiply : Product  Multiplication=Matrix(*)
  Quaternion to Euler Angles : QuaternionLibrary/Quaternion to Euler Angles
  Scope : Scope
  Selector : Selector  InputPortWidth=3  IndexOptions=Index vector (dialog)  Indices=3  OutputSizes=1
  " horThrustBody" : Outport  VectorParamsAs1DForOutWhenUnconnected=off
  wires:
  Matrix Multiply/1 -> " horThrustBody"/1
  2D Rotation Matrix/1(R) -> Matrix Multiply/1
  "q "/1 -> Quaternion to Euler Angles/1
  Selector/1 -> Scope/1, 2D Rotation Matrix/1(psi)
  Quaternion to Euler Angles/1 -> Selector/1
  "horThrust "/1 -> Matrix Multiply/2

== system MultirotorSimPx4v1_8FPHTFullGainMatrix/Pos Control/Rotation/2D Rotation Matrix ==
  psi : Inport
  Cos : Trigonometry  Operator=cos
  Display : Display
  Gain : Gain  Gain=-1
  Matrix Concatenate : Concatenate  Mode=Multidimensional array  ConcatenateDimension=2
  Mux : Mux  Inputs=2
  Mux1 : Mux  Inputs=2
  Sin : Trigonometry
  R : Outport  VectorParamsAs1DForOutWhenUnconnected=off
  wires:
  Cos/1 -> Mux1/2, Mux/1
  Sin/1 -> Mux1/1, Gain/1
  Mux/1 -> Matrix Concatenate/1
  Gain/1 -> Mux/2
  Mux1/1 -> Matrix Concatenate/2
  Matrix Concatenate/1 -> Display/1, R/1
  psi/1 -> Sin/1, Cos/1

== system MultirotorSimPx4v1_8FPHTFullGainMatrix/Pos Control1/Rotation/2D Rotation Matrix ==
  psi : Inport
  Cos : Trigonometry  Operator=cos
  Display : Display
  Gain : Gain  Gain=-1
  Matrix Concatenate : Concatenate  Mode=Multidimensional array  ConcatenateDimension=2
  Mux : Mux  Inputs=2
  Mux1 : Mux  Inputs=2
  Sin : Trigonometry
  R : Outport  VectorParamsAs1DForOutWhenUnconnected=off
  wires:
  Cos/1 -> Mux1/2, Mux/1
  Sin/1 -> Mux1/1, Gain/1
  Mux/1 -> Matrix Concatenate/1
  Gain/1 -> Mux/2
  Mux1/1 -> Matrix Concatenate/2
  Matrix Concatenate/1 -> Display/1, R/1
  psi/1 -> Sin/1, Cos/1

== matlab function MultirotorSimPx4v1_8FPHTFullGainMatrix/Compute Sph ==
  data: in input; beta output; alpha output; R output
function [beta, alpha, R] = computeSph(in)
%#codegen

% Convert from polar to spherical coordinates
[ beta, alpha, R ] = cart2sph( in(1), in(2), in(3) );

== matlab function MultirotorSimPx4v1_8FPHTFullGainMatrix/Quadrotor Euler Model/Compute etaDot ==
  data: nuBody input; eta input; etaDot output
function etaDot = computeEtaDot(nuBody, eta)
%#codegen

sPhi = sin(eta(1));
cPhi = cos(eta(1));
cTheta = cos(eta(2));
tTheta = tan(eta(2));
      
WInverse = [1, sPhi*tTheta,  cPhi*tTheta;
            0, cPhi,        -sPhi;
            0, sPhi/cTheta,  cPhi/cTheta];

etaDot = WInverse*nuBody;

== matlab function MultirotorSimPx4v1_8FPHTFullGainMatrix/Quadrotor Euler Model/compute VBody ==
  data: eta input; VBody output; xiDot input
function VBody = computeVBody(eta, xiDot)
%#codegen

sphi = sin(eta(1));
sTheta = sin(eta(2));
sPsi = sin(eta(3));
cPhi = cos(eta(1));
cTheta = cos(eta(2));
cPsi = cos(eta(3));

R = [ cPsi*cTheta, cPsi*sTheta*sphi-sPsi*cPhi, cPsi*sTheta*cPhi+sPsi*sphi;
	  sPsi*cTheta, sPsi*sTheta*sphi+cPsi*cPhi, sPsi*sTheta*cPhi-cPsi*sphi;
     -sTheta,      cTheta*sphi,                cTheta*cPhi+sPsi*sphi];

VBody = R'*xiDot;

== matlab function MultirotorSimPx4v1_8FPHTFullGainMatrix/L2 norm ==
  data: u input; y output
function y = l2norm( u )
    y = sqrt( dot(u, u) );
end

== matlab function MultirotorSimPx4v1_8FPHTFullGainMatrix/Motor model 2/Compute Sph ==
  data: V_appBody input; polar output
function polar  = computeSph(V_appBody)
%#codegen

% Convert from polar to spherical coordinates
[ azimuth, elevation, radius ] = cart2sph( V_appBody(1), V_appBody(2), V_appBody(3) );

polar = [azimuth; elevation; radius];

== matlab function MultirotorSimPx4v1_8FPHTFullGainMatrix/Motor model 2/Individual motor force//torque ==
  data: omega input; TMotorIndividual output; omegaDot input; polarC input; Motor parameter; Uav parameter; tauMotorIndividual output; Aero parameter
function [TMotorIndividual, tauMotorIndividual] = motorIndividual( ...
    omega, omegaDot, polarC, Motor, Uav, Aero)
%#codegen
    alpha = polarC(2);
    beta  = polarC(1);
    U     = polarC(3);

    % Make assertions to avoid code generation errors
    %assert(Uav.N_ROTORS < 16);
    % Uav.N_ROTORS = 4;

    % Output
    % TMotorIndividual   = zeros(3, Uav.N_ROTORS);
    %tauMotorIndividual = zeros(3, Uav.N_ROTORS);

    %% Thrust and differential torque

    % Concatenated motor force/torque vectors in respective motor frame
    % eg. TMotor = [TMotor1, TMotor2, ..., TMotorN]
    % where: - N is the number of rotors
    %        - TMotorx (x ∈ [1,2,...,N]) is the thrust generated by motor x in
    %          its own frame of reference
    % For basic thrust model:
    % TMotorIndividual = [ zeros(2, Uav.N_ROTORS);
    %                      K * (omega'.^2) ];

    Cz2 = dot( Aero.Cz2.coefs, [alpha, 1]);
    p = Aero.Cz3.coefs;
    lambda = omega .* Uav.D_PROP / ( 2 * U );
    Cz3 = p(1) * sin(alpha) + p(2) * ( 1 - exp(-p(3).*lambda) ) .* sin(3*alpha) + ...
        p(4);
    p = Aero.Cx2.coefs;
    Cx2 = p(1) * ( 1 - exp(-p(2).*lambda) ) .* cos(alpha) + ...
          p(3) * ( 1 - exp(-p(4).*lambda) ) .* cos(3*alpha);
    Tz = -0.5 .* Uav.RHO_AIR .* omega'.^2 .* (Cz2) .* Uav.D_PROP^2 .* Uav.A_PROP - ... % Rotor thrust
          0.5 .* Uav.RHO_AIR .* (Cz3)' .* U .*  omega' .* Uav.D_PROP .* Uav.A_PROP;    % Rotor thrust correction
    Tx = -0.5 .* Uav.RHO_AIR .* (Cx2)' .* U .* omega' .* Uav.D_PROP .* Uav.A_PROP;
    TMotorIndividual = [ Tx.*cos(beta); Tx.*sin(beta); Tz ];

    tauMotorIndividual = [ 0*omega'; 0*omega'; % Avoid using zeros(1,Uav.N_ROTORS), which causes issues
        -Uav.ROTOR_DIRECTION .* ( Motor.B .* omega'.^2 + Motor.I_R_ZZ .* omegaDot' ) ];
end

== matlab function MultirotorSimPx4v1_8FPHTFullGainMatrix/Motor model 2/Combined motor force//torque ==
  data: TMotorIndividual input; TBody output size=3; tauMotorIndividual input; tauBody output size=3; omega input; nuBody input; Motor parameter; Uav parameter
function [TBody, tauBody] = motorCombined( TMotorIndividual,tauMotorIndividual,  ...
    omega, nuBody, Motor, Uav)
%#codegen
assert(Uav.N_ROTORS < 16);

% Initialise matrices to store motor force/torque vectors in body frame
TBodyIndividual   = zeros(3, Uav.N_ROTORS);
tauBodyIndividual = zeros(3, Uav.N_ROTORS);

% Calculate forces and moments from each motor in the body frame
for i = 1:Uav.N_ROTORS
    l = Uav.L(i);
    beta = Uav.BETA(i);
    
    % Matrix to compute torque applied by rotor thrust
 	L = [ 0,            0,            l*sin(beta);
          0,            0,           -l*cos(beta);
         -l*sin(beta),  l*cos(beta),  0 ];

	% Motor force/torque vectors in body frame
	TBodyIndividual(:,i) = Uav.R_MOTOR_TO_BODY(:,:,i) * ...
        TMotorIndividual(:,i);
	tauBodyIndividual(:,i) = Uav.R_MOTOR_TO_BODY(:,:,i) * ...
        tauMotorIndividual(:,i) + L * TBodyIndividual(:,i);
end

%% Gyroscopic moments

% Concatenated gyroscopic moments for each rotor
M_GBodyIndividual = zeros(3, Uav.N_ROTORS);
H_MMotorSeparate = zeros(3, Uav.N_ROTORS);

% Concatenated motor speeds in their respective frames
omegaMotor = [ zeros(2, Uav.N_ROTORS);
               Uav.ROTOR_DIRECTION .* omega' ];

for i = 1:Uav.N_ROTORS
    % Angular momentum in motor frame
    H_MMotorSeparate(:,i) = Motor.I_R(:,:,i) * omegaMotor(:,i);
    % Gyroscopic moment vectors in body frame
    M_GBodyIndividual(:,i) = cross( nuBody, ...
        Uav.R_MOTOR_TO_BODY(:,:,i) * H_MMotorSeparate(:,i) );
end

M_GBody = sum(M_GBodyIndividual, 2);

%% Total torque and moment

% Total force/torque in body frame
TBody = sum(TBodyIndividual, 2);
tauBody = sum(tauBodyIndividual, 2) - M_GBody;

end

== matlab function MultirotorSimPx4v1_8FPHTFullGainMatrix/Motor model 2/Motor rotational dynamics ==
  data: pwm input; omegaDot output; omega input; realPwm output
function [omegaDot, realPwm]  = motorRotDynamics( pwm, omega )
%#codegen

realPwm = (1000 * pwm + 1000);

rotorTimeConst = 7.006512e-02;
omegaRef = 0.84 * ( 7.969173e-1.*realPwm - 6.528579e2 );

omegaDot = (omegaRef - omega) / rotorTimeConst;
end

== matlab function MultirotorSimPx4v1_8FPHTFullGainMatrix/Quadrotor Euler Model/Equations of motion ==
  data: VBody input; VBodyDot output; nuBody input; eta input; etaDot input; TBody input size=3; tauBody input size=3; F_D input size=3; M_D input size=3; nuBodyDot output; Uav parameter; xiDDot output; etaDDot output
function [VBodyDot, nuBodyDot, xiDDot, etaDDot] = QuadrotorQuaternionModel(...
    VBody, nuBody, eta, etaDot, TBody, tauBody, F_D, M_D, Uav )
%#codegen

%% Rotation matrices
% Precompute sines and cosines
sPhi   = sin(eta(1));
sTheta = sin(eta(2));
sPsi   = sin(eta(3));
cPhi   = cos(eta(1));
cTheta = cos(eta(2));
cPsi   = cos(eta(3));
tTheta = tan(eta(2));

phiDot   = etaDot(1);
thetaDot = etaDot(2);

% Body frame to inertial frame
R = [cPsi*cTheta, cPsi*sTheta*sPhi-sPsi*cPhi, cPsi*sTheta*cPhi+sPsi*sPhi;
     sPsi*cTheta, sPsi*sTheta*sPhi+cPsi*cPhi, sPsi*sTheta*cPhi-cPsi*sPhi;
     -sTheta,     cTheta*sPhi,                cTheta*cPhi+sPsi*sPhi];

WInvertDot = [...
    0,  phiDot*cPhi*tTheta+thetaDot*sPhi/cTheta^2,    -phiDot*sPhi*cTheta+thetaDot*cPhi/cTheta^2;
    0, -phiDot*sPhi,                                  -phiDot*cPhi;
	0,  phiDot*cPhi/cTheta+phiDot*sPhi*tTheta/cTheta, -phiDot*sPhi/cTheta+thetaDot*cPhi*tTheta/cTheta];

WInvert = [1, sPhi*tTheta,  cPhi*tTheta;
           0, cPhi,        -sPhi;
           0, sPhi/cTheta,  cPhi/cTheta];


%% Moments and Forces
% Body frame accelerations
VBodyDot  = (1/Uav.M) * (R'*Uav.G + TBody - cross(nuBody, Uav.M*VBody) + F_D);
nuBodyDot = Uav.I \ (tauBody - cross(nuBody, Uav.I*nuBody) + M_D);

% Inertial frame accelerations
xiDDot = (1/Uav.M)*(Uav.G + R*TBody + R*F_D);
etaDDot = WInvertDot*nuBody + WInvert*nuBodyDot;

end

== matlab function MultirotorSimPx4v1_8FPHTFullGainMatrix/Pos Control1/MATLAB Function ==
  data: thr_sp input size=3; q_sp output; yaw_sp input; thrust_sp output
function [q_sp, thrust_sp] = thrustToAttitude( thr_sp, yaw_sp )

    yaw_body = yaw_sp;
    body_z = -thr_sp./norm(thr_sp);
    
    y_C = [ -sin(yaw_body); cos(yaw_body); 0 ];
    
    body_x = zeros(3,1);
    if body_z(3) > 0.000001
        body_x = cross( y_C, body_z );
        if ( body_z(3) < 0 )
            body_x = -body_x;
        end
        
        body_x = body_x ./ norm(body_x);
    else
        body_x(3) = 1;
    end
    
    body_y = cross( body_z, body_x );
    
    R_sp = [ body_x, body_y, body_z ];
    
    q_sp = from_dcm( R_sp );
    
    thrust_sp = -norm( thr_sp );
    
end

function data  = from_dcm( dcm )
% FROM_DCM Convert DCM to quaternion
% From https://github.com/PX4/Firmware/blob/master/src/lib/mathlib/math/Quaternion.hpp
    data = zeros(4,1);
    tr = dcm(1,1) + dcm(2,2) + dcm(3,3);
    if (tr > 0.0)
        s = sqrt(tr + 1.0);
        data(1) = s * 0.5;
        s = 0.5 / s;
        data(2) = (dcm(3,2) - dcm(2,3) ) * s;
        data(3) = (dcm(1,3) - dcm(3,1) ) * s;
        data(4) = (dcm(2,1) - dcm(1,2) ) * s;
    else
        % Find maximum diagonal element in dcm
        % store index in dcm_i
        dcm_i = 1;
        for i = 2:3 % (int i = 1; i < 3; i++)
            if ( dcm(i,i) > dcm(dcm_i,dcm_i) )
                dcm_i = i;
            end
        end
        dcm_j = rem( ( (dcm_i-1) + 1), 3) + 1;
        dcm_k = rem( ( (dcm_i-1) + 2), 3) + 1;
        s = sqrt( (dcm(dcm_i, dcm_i) - dcm(dcm_j, dcm_j) - ...
            dcm(dcm_k,dcm_k)) + 1.0 );
        data(dcm_i + 1) = s * 0.5;
        s = 0.5 / s;
        data(dcm_j + 1) = ( dcm(dcm_i,dcm_j) + dcm(dcm_j,dcm_i) ) * s;
        data(dcm_k + 1) = ( dcm(dcm_k,dcm_i) + dcm(dcm_i,dcm_k) ) * s;
        data(1) = ( dcm(dcm_k,dcm_j) - dcm(dcm_j,dcm_k) ) * s;
    end
end

== matlab function MultirotorSimPx4v1_8FPHTFullGainMatrix/Pos Control/MATLAB Function1 ==
  data: thr_sp input size=3; q_sp output; yaw_sp input; thrust_sp output
function [q_sp, thrust_sp] = thrustToAttitude( thr_sp, yaw_sp )

    yaw_body = yaw_sp;
    body_z = -thr_sp./norm(thr_sp);
    
    y_C = [ -sin(yaw_body); cos(yaw_body); 0 ];
    
    body_x = zeros(3,1);
    if body_z(3) > 0.000001
        body_x = cross( y_C, body_z );
        if ( body_z(3) < 0 )
            body_x = -body_x;
        end
        
        body_x = body_x ./ norm(body_x);
    else
        body_x(3) = 1;
    end
    
    body_y = cross( body_z, body_x );
    
    R_sp = [ body_x, body_y, body_z ];
    
    q_sp = from_dcm( R_sp );
    
    thrust_sp = -norm( thr_sp );
    
end

function data  = from_dcm( dcm )
% FROM_DCM Convert DCM to quaternion
% From https://github.com/PX4/Firmware/blob/master/src/lib/mathlib/math/Quaternion.hpp
    data = zeros(4,1);
    tr = dcm(1,1) + dcm(2,2) + dcm(3,3);
    if (tr > 0.0)
        s = sqrt(tr + 1.0);
        data(1) = s * 0.5;
        s = 0.5 / s;
        data(2) = (dcm(3,2) - dcm(2,3) ) * s;
        data(3) = (dcm(1,3) - dcm(3,1) ) * s;
        data(4) = (dcm(2,1) - dcm(1,2) ) * s;
    else
        % Find maximum diagonal element in dcm
        % store index in dcm_i
        dcm_i = 1;
        for i = 2:3 % (int i = 1; i < 3; i++)
            if ( dcm(i,i) > dcm(dcm_i,dcm_i) )
                dcm_i = i;
            end
        end
        dcm_j = rem( ( (dcm_i-1) + 1), 3) + 1;
        dcm_k = rem( ( (dcm_i-1) + 2), 3) + 1;
        s = sqrt( (dcm(dcm_i, dcm_i) - dcm(dcm_j, dcm_j) - ...
            dcm(dcm_k,dcm_k)) + 1.0 );
        data(dcm_i + 1) = s * 0.5;
        s = 0.5 / s;
        data(dcm_j + 1) = ( dcm(dcm_i,dcm_j) + dcm(dcm_j,dcm_i) ) * s;
        data(dcm_k + 1) = ( dcm(dcm_k,dcm_i) + dcm(dcm_i,dcm_k) ) * s;
        data(1) = ( dcm(dcm_k,dcm_j) - dcm(dcm_j,dcm_k) ) * s;
    end
end

== matlab function MultirotorSimPx4v1_8FPHTFullGainMatrix/Applied wind speed/Relative velocity ==
  data: nuBody input; Uav parameter; VMotorRelBody output
function VMotorRelBody = relativeMotorVelocity( nuBody , Uav )
%#codegen
    VMotorRelBody = cross( nuBody, Uav.L_VEC );
end

== matlab function MultirotorSimPx4v1_8FPHTFullGainMatrix/Applied wind speed/Compute V_app2 ==
  data: Q input; UBody output; U input size=3
function UBody = computeUBody(Q, U)
%#codegen

% Rotation matrix from Wind frame to Inertial frame
% Wind frame SEU, inertial frame NED
R_U = [1,  0, 0;
       0, -1, 0;
       0,  0, 1];
   
UBody = Q' * R_U * U;
